simulink model "LCK_AVP"  (R2018b)
settings: Solver=FixedStepDiscrete  StartTime=0.0  StopTime=inf  FixedStep=0.01  RelTol=1e-3
PreLoadFcn:
  | if exist('tl_preloadfcn','file'), tl_preloadfcn(gcs,'4.4.0.41'); end
PostLoadFcn:
  | if any(exist('dsrtsu_mdlpostloadfcn', 'file') ~= 0), dsrtsu_mdlpostloadfcn('Execute', bdroot); end
  | if exist('tl_postloadfcn','file'), tl_postloadfcn(gcs,'4.4.0.41'); end
InitFcn:
  | if exist('tlds_init','file'), tlds_init(gcs); end
StartFcn:
  | if exist('tlds_start','file'), tlds_start(gcs); end
StopFcn:
  | if exist('tlds_stop','file'), tlds_stop(gcs); end
values from neighbouring files (symbols this model uses):
  C_DEG2RAD = 0.0175    [LCK_Macro.sldd]
  C_KPH2MPS = 0.2778    [LCK_Macro.sldd]
  C_NEARZERO = 0.0001    [LCK_Macro.sldd]
  C_ONE = 1.0    [LCK_Macro.sldd]
  C_RAD2DEG = 57.2958    [LCK_Macro.sldd]
  C_ZERO = 0.0    [LCK_Macro.sldd]
  k_accel_pedal_pos_per_speed_x : value not decoded    [LCK_LogicPara.sldd]
  k_accel_pedal_pos_per_speed_z : value not decoded    [LCK_LogicPara.sldd]
  k_brake_suprress_hold = 1000.0    [LCK_LogicPara.sldd]
  k_driver_appl_torque_filt = 50.0    [LCK_LogicPara.sldd]
  k_driver_suppression_hold_time = 3000.0    [LCK_LogicPara.sldd]
  k_hands_on_wheel_hold_msec = 500.0    [LCK_LogicPara.sldd]
  k_hands_on_wheel_torque_hi = 0.2    [LCK_LogicPara.sldd]
  k_hands_on_wheel_torque_lo = 0.15    [LCK_LogicPara.sldd]
  k_handsoff_delay_cycles = 50.0    [LCK_LogicPara.sldd]
  k_handsoff_torq_Lo_CR = 0.3    [LCK_LogicPara.sldd]
  k_handson_delay_cycles = 5.0    [LCK_LogicPara.sldd]
  k_HighAccel_suppress_hold = 3000.0    [LCK_LogicPara.sldd]
  k_HLR_suprress_hold = 3000.0    [LCK_LogicPara.sldd]
  k_hs_StrAng_CR_threshold_z : value not decoded    [LCK_LogicPara.sldd]
  k_LC_Exit_Switch = 0.0    [LCK_LogicPara.sldd]
  k_LCG_Configured = 1.0    [LCK_LogicPara.sldd]
  k_LCK_A0_Rdy2Act_UseConst = 0.0    [LCK_LogicPara.sldd]
  k_LCK_A0Fac_ActSta : value not decoded    [LCK_CtrlPara.sldd]
  k_LCK_A0Fac_DrvStm : value not decoded    [LCK_CtrlPara.sldd]
  k_LCK_A0Shift_LftCurv : value not decoded    [LCK_CtrlPara.sldd]
  k_LCK_A0Shift_RgtCurv : value not decoded    [LCK_CtrlPara.sldd]
  k_LCK_A0Shift_StraLan = 0.0    [LCK_CtrlPara.sldd]
  k_LCK_A0ShiftFac_Dy_LftCurv : value not decoded    [LCK_CtrlPara.sldd]
  k_LCK_A0ShiftFac_Dy_RgtCurv : value not decoded    [LCK_CtrlPara.sldd]
  k_LCK_A0ShiftFac_Vspd : value not decoded    [LCK_CtrlPara.sldd]
  k_LCK_accel_inhibit_thold = 35.0    [LCK_LogicPara.sldd]
  k_LCK_Active2Ready_Mask = 255.0    [LCK_LogicPara.sldd]
  k_LCK_CvatRateBks : value not decoded    [LCK_CtrlPara.sldd]
  k_LCK_CvatrBks : value not decoded    [LCK_CtrlPara.sldd]
  k_LCK_DFac_Dy : value not decoded    [LCK_CtrlPara.sldd]
  k_LCK_DFac_Dy_Curv : value not decoded    [LCK_CtrlPara.sldd]
  k_LCK_DFac_HaCurCen : value not decoded    [LCK_CtrlPara.sldd]
  k_LCK_DFac_HaCurSid : value not decoded    [LCK_CtrlPara.sldd]
  k_LCK_DFac_HadCurCen : value not decoded    [LCK_CtrlPara.sldd]
  k_LCK_DFac_HadCurSid : value not decoded    [LCK_CtrlPara.sldd]
  k_LCK_DFac_HadStrCen : value not decoded    [LCK_CtrlPara.sldd]
  k_LCK_DFac_HadStrSid : value not decoded    [LCK_CtrlPara.sldd]
  k_LCK_DFac_HaStrCen : value not decoded    [LCK_CtrlPara.sldd]
  k_LCK_DFac_HaStrSid : value not decoded    [LCK_CtrlPara.sldd]
  k_LCK_DFac_Rad : value not decoded    [LCK_CtrlPara.sldd]
  k_LCK_DFac_SA_CurCen : value not decoded    [LCK_CtrlPara.sldd]
  k_LCK_DFac_SA_CurSid : value not decoded    [LCK_CtrlPara.sldd]
  k_LCK_DFac_SA_StrCen : value not decoded    [LCK_CtrlPara.sldd]
  k_LCK_DFac_SA_StrSid : value not decoded    [LCK_CtrlPara.sldd]
  k_LCK_DFac_SS_CurCen : value not decoded    [LCK_CtrlPara.sldd]
  k_LCK_DFac_SS_CurSid : value not decoded    [LCK_CtrlPara.sldd]
  k_LCK_DFac_SS_StrCen : value not decoded    [LCK_CtrlPara.sldd]
  k_LCK_DFac_SS_StrSid : value not decoded    [LCK_CtrlPara.sldd]
  k_LCK_DFac_Vspd : value not decoded    [LCK_CtrlPara.sldd]
  k_LCK_DlyTm_DrvStim = 0.2    [LCK_CtrlPara.sldd]
  k_LCK_DTermMax = 2.0    [LCK_CtrlPara.sldd]
  k_LCK_DyBks_Curv : value not decoded    [LCK_CtrlPara.sldd]
  k_LCK_Enable_POOnly = 1.0    [LCK_LogicPara.sldd]
  k_LCK_Entry_DistBuffer = 0.1    [LCK_LogicPara.sldd]
  k_LCK_Fac_Vspd2RngThr_FalRec = 0.23    [LCK_CtrlPara.sldd]
  k_LCK_Ffw_CvatSwh = 0.0    [LCK_CtrlPara.sldd]
  k_LCK_Ffw_DyBks : value not decoded    [LCK_CtrlPara.sldd]
  k_LCK_Ffw_TimCon_CmdFlt = 0.0    [LCK_CtrlPara.sldd]
  k_LCK_FfwDeltaFac_Rad_Lft : value not decoded    [LCK_CtrlPara.sldd]
  k_LCK_FfwDeltaFac_Rad_Rgt : value not decoded    [LCK_CtrlPara.sldd]
  k_LCK_FfwDeltaFac_Vspd : value not decoded    [LCK_CtrlPara.sldd]
  k_LCK_FfwFac_CvatRate_Lft : value not decoded    [LCK_CtrlPara.sldd]
  k_LCK_FfwFac_CvatRate_Rgt : value not decoded    [LCK_CtrlPara.sldd]
  k_LCK_FfwFac_Dy : value not decoded    [LCK_CtrlPara.sldd]
  k_LCK_FfwFac_Rad_Lft : value not decoded    [LCK_CtrlPara.sldd]
  k_LCK_FfwFac_Rad_Rgt : value not decoded    [LCK_CtrlPara.sldd]
  k_LCK_FfwFac_Vspd : value not decoded    [LCK_CtrlPara.sldd]
  k_LCK_FfwTorq_Cvat : value not decoded    [LCK_CtrlPara.sldd]
  k_LCK_HAFac_ActSta : value not decoded    [LCK_CtrlPara.sldd]
  k_LCK_HAFac_DrvStm : value not decoded    [LCK_CtrlPara.sldd]
  k_LCK_HaloTime = 2000.0    [LCK_LogicPara.sldd]
  k_LCK_HaloTime_Switch = 0.0    [LCK_LogicPara.sldd]
  k_LCK_HARFac_ActSta : value not decoded    [LCK_CtrlPara.sldd]
  k_LCK_HARFac_DrvStm : value not decoded    [LCK_CtrlPara.sldd]
  k_LCK_Hed_DyBks : value not decoded    [LCK_CtrlPara.sldd]
  k_LCK_HedAngDiffX : value not decoded    [LCK_CtrlPara.sldd]
  k_LCK_HedAngRateDiffX : value not decoded    [LCK_CtrlPara.sldd]
  k_LCK_HndsOnWhel_DlyTm_Idl2Rdy = 0.0    [LCK_LogicPara.sldd]
  k_LCK_host_veh_width = 1.86    [LCK_LogicPara.sldd]
  k_LCK_Idle2Ready_Mask = 239.0    [LCK_LogicPara.sldd]
  k_LCK_Junc_SusTime = 1.0    [LCK_LogicPara.sldd]
  k_LCK_KpKdDecSlopeLmt = 10.0    [LCK_CtrlPara.sldd]
  k_LCK_KpKdIncSlopeLmt = 5.0    [LCK_CtrlPara.sldd]
  k_LCK_Lat_Ctrl_DFac_Lft = 1.0    [LCK_CtrlPara.sldd]
  k_LCK_Lat_Ctrl_DFac_Rgt = 1.05    [LCK_CtrlPara.sldd]
  k_LCK_Lat_Ctrl_Kd = 0.8    [LCK_CtrlPara.sldd]
  k_LCK_Lat_Ctrl_Ki = 0.5    [LCK_CtrlPara.sldd]
  k_LCK_Lat_Ctrl_Kp = 0.7    [LCK_CtrlPara.sldd]
  k_LCK_Lat_Ctrl_Kp_NearGain = 0.7    [LCK_CtrlPara.sldd]
  k_LCK_Lat_Ctrl_PFac_Lft = 1.0    [LCK_CtrlPara.sldd]
  k_LCK_Lat_Ctrl_PFac_Rgt = 1.05    [LCK_CtrlPara.sldd]
  k_LCK_Lat_Ctrl_TimCon_CmdFlt = 5.0    [LCK_CtrlPara.sldd]
  k_LCK_Lat_DFac_Rad : value not decoded    [LCK_CtrlPara.sldd]
  k_LCK_Lat_DFac_SS_Cur : value not decoded    [LCK_CtrlPara.sldd]
  k_LCK_Lat_DFac_SS_Str : value not decoded    [LCK_CtrlPara.sldd]
  k_LCK_Lat_DFac_Vspd : value not decoded    [LCK_CtrlPara.sldd]
  k_LCK_Lat_DyBks : value not decoded    [LCK_CtrlPara.sldd]
  k_LCK_Lat_IFac_Rad : value not decoded    [LCK_CtrlPara.sldd]
  k_LCK_Lat_IFac_Vspd : value not decoded    [LCK_CtrlPara.sldd]
  k_LCK_Lat_ILmtFac_Dy_CurvLan : value not decoded    [LCK_CtrlPara.sldd]
  k_LCK_Lat_ILmtFac_Dy_StraLan : value not decoded    [LCK_CtrlPara.sldd]
  k_LCK_Lat_ILmtFac_Rad : value not decoded    [LCK_CtrlPara.sldd]
  k_LCK_Lat_ILmtFac_Rad_NearGain = 1.0    [LCK_CtrlPara.sldd]
  k_LCK_Lat_ILmtFac_Vspd_CurvLan : value not decoded    [LCK_CtrlPara.sldd]
  k_LCK_Lat_ILmtFac_Vspd_StraLan : value not decoded    [LCK_CtrlPara.sldd]
  k_LCK_Lat_ITermLmt_Dy = 1.0    [LCK_CtrlPara.sldd]
  k_LCK_Lat_KpKdDecSlopeLmt = 10.0    [LCK_CtrlPara.sldd]
  k_LCK_Lat_KpKdIncSlopeLmt = 10.0    [LCK_CtrlPara.sldd]
  k_LCK_Lat_PFac_Dy_InnLftCur : value not decoded    [LCK_CtrlPara.sldd]
  k_LCK_Lat_PFac_Dy_InnRgtCur : value not decoded    [LCK_CtrlPara.sldd]
  k_LCK_Lat_PFac_Dy_OutLftCur : value not decoded    [LCK_CtrlPara.sldd]
  k_LCK_Lat_PFac_Dy_OutRgtCur : value not decoded    [LCK_CtrlPara.sldd]
  k_LCK_Lat_PFac_Dy_Str : value not decoded    [LCK_CtrlPara.sldd]
  k_LCK_Lat_PFac_Rad : value not decoded    [LCK_CtrlPara.sldd]
  ... (+153 more)
undefined symbols (not defined in the file or in its folder): k_LCK_CurvBks, K_LCK_SPA0A1A2_LMRngCmp_y
libraries: LateralControl_fcns_lib x58, simulink x24
(part 25 of 48)

== system LCK_AVP/Lateral_Control_Module/LCK_State_Ctrl/Det_Driver_Operation/Det_Driver_Steer_Override ==
  note: Pos = driver steers left
  note: Detect driver override during left lane marker intervention:
      | auto steer right + driver torque point left = f_driver_override
  note: Detect driver override during right lane marker intervention:
      | auto steer left + driver torque point right = f_driver_override
  note: Determine Driver Steering Override
  note: Steer angle rate: pos = velocity left
      | neg = velocity right
  note: Steer_angle: positive = left, CCW
      | negative= right,CW
  LCK_Mode : Inport  Description=_GWMAB30P4.LCK.000_38_
  Final_Torq_Cmd : Inport  Description=_GWMAB30P4.LCK.000_39_  Port=2
  Vspd : Inport  Description=_GWMAB30P4.LCK.000_38_  Port=3
  Steer_Torq : Inport  Description=_GWMAB30P4.LCK.000_38_  Port=4
  Add : Sum  Tag={'output',{'type','Float32'},'date',737395.45720195607}  Description=_GWMH9P3.LCK.000_11_  Inputs=-+
  Constant : Constant  Tag={'output',{'type','Int32'},'date',737237.63745600695}  Description=_GWMAB30P3.LCK.000_10_  Value=0
  Constant1 : Constant  Tag={'output',{'type','Int32'},'date',737237.63745672454}  Description=_GWMAB30P3.LCK.000_11_  Value=0
  Constant10 : Constant  Tag={'output',{'name','$P','class','EXTERN_CAL','type','Float32'},'date',737246.86422390048}  Description=_GWMAB30P2.LCK.000_1019_  Value=k_override_right_torq_thold
  Constant14 : Constant  Tag={'output',{'name','$P','class','EXTERN_CAL','type','Bool'},'date',737246.86427055555}  Description=_GWMAB30P2.LCK.000_1022_  Value=k_Ovrd_torq_thold_per_spd_sw
  Constant15 : Constant  Tag={'output',{'name','$P','class','EXTERN_CAL','type','Bool'},'date',737246.86427074077}  Description=_GWMAB30P2.LCK.000_1023_  Value=k_Ovrd_torq_thold_per_spd_sw
  Constant7 : Constant  Tag={'output',{'name','$P','class','EXTERN_CAL','type','Float32'},'date',737246.86422540504}  Description=_GWMAB30P2.LCK.000_1027_  Value=k_override_left_torq_thold
  Data Type Conversion1 : DataTypeConversion  Description=_GWMAB30P4.LCK.000_40_
  Data Type Conversion3 : DataTypeConversion  Description=_GWMAB30P4.LCK.000_41_
  Data Type Conversion4 : DataTypeConversion  Description=_GWMAB30P4.LCK.000_42_
  Data Type Conversion8 : DataTypeConversion  Description=_GWMAB30P4.LCK.000_43_
  Delay : Delay  DelayLength=1  InitialCondition=0
  Delay1 : Delay  DelayLength=1  InitialCondition=0
  Gain : Gain  Tag={'output',{'type','Float32'},'gain',{'type','Int32'},'date',737189.64304143516}  Description=_GWMAB30P2.LCK.000_1028_  Gain=-1
  Logical Operator : Logic  Tag={'date',737237.63745719905}  Description=_GWMAB30P3.LCK.000_12_  AllPortsSameDT=off  OutDataTypeStr=boolean
  Logical Operator1 : Logic  Tag={'date',737237.63745734957}  Description=_GWMAB30P3.LCK.000_13_  AllPortsSameDT=off  OutDataTypeStr=boolean
  Logical Operator2 : Logic  Tag={'date',737393.53532744211}  Description=_GWMH9P3.LCK.000_12_  Operator=OR  AllPortsSameDT=off  OutDataTypeStr=boolean
  Relational Operator : RelationalOperator  Tag={'date',737237.63745749998}  Description=_GWMAB30P3.LCK.000_14_  Operator=<  OutDataTypeStr=boolean  RndMeth=Nearest
  Relational Operator1 : RelationalOperator  Tag={'date',737237.63745763886}  Description=_GWMAB30P3.LCK.000_15_  Operator=>  OutDataTypeStr=boolean  RndMeth=Nearest
  Relational Operator3 : RelationalOperator  Tag={'date',737184.60396784719}  Description=_GWMAB30P2.LCK.000_1039_  OutDataTypeStr=boolean  RndMeth=Nearest
  Relational Operator6 : RelationalOperator  Tag={'date',737184.60396796302}  Description=_GWMAB30P2.LCK.000_1040_  Operator=<=  OutDataTypeStr=boolean  RndMeth=Nearest
  Right_distance_sustain_period : Stateflow chart  Description=_GWMAB30P4.LCK.000_44_  TreatAsAtomicUnit=on
  Switch : Switch  Tag={'output',{'inheritscaling',1},'threshold',{'type','Int32','scalar',1},'date',737395.45749100694}  Description=_GWMH9P3.LCK.000_13_  Criteria=u2 ~= 0
  Switch2 : Switch  Tag={'output',{'inheritscaling',1},'threshold',{'type','Int32','scalar',1},'date',737189.6437576852}  Description=_GWMAB30P2.LCK.000_1045_  Threshold=0.5
  Switch3 : Switch  Tag={'output',{'inheritscaling',1},'threshold',{'type','Int32','scalar',1},'date',737189.64308021986}  Description=_GWMAB30P2.LCK.000_1046_  Threshold=0.5
  Unit Delay1 : UnitDelay  Tag={'output',{'inheritscaling',1},'state',{'type','Int32'},'date',737395.45284084487}  Description=_GWMH9P3.LCK.000_14_  SampleTime=-1
  Unit Delay2 : UnitDelay  Tag={'output',{'inheritscaling',1},'state',{'type','Int32'},'date',737395.45284105325}  Description=_GWMH9P3.LCK.000_15_  SampleTime=-1
  k_LCK_Ovrd_Torq_Hys : Constant  Tag={'output',{'name','$P','class','EXTERN_CAL','type','Float32'},'date',737395.45723880793}  Description=_GWMH9P3.LCK.000_16_  Value=k_LCK_Ovrd_Torq_Hys
  k_LCK_ovrd_torq_thold_per_spd : Lookup_n-D  Tag={'input',{'name','$P','class','EXTERN_CAL','type','Float32'},'output',{'type','Float32'},'table',{'name','$P','class','EXTERN_CAL','type','Float32'},'date',737237.77625888889}  Description=_GWMAB30P2.LCK.000_1047_  NumberOfTableDimensions=1  BreakpointsForDimension1=k_LCK_ovrd_torq_thold_per_spd_x  IndexSearchMethod=Linear search  Table=k_LCK_ovrd_torq_thold_per_spd_z  ExtrapMethod=Clip  InputSameDT=on
  left_distance_sustain_period : Stateflow chart  Description=_GWMAB30P4.LCK.000_49_  TreatAsAtomicUnit=on
  within_distance_sustain_period : Constant  Tag={'output',{'name','$P','class','EXTERN_CAL','type','UInt16'},'date',737246.8642231134}  Description=_GWMAB30P2.LCK.000_1051_  Value=k_override_torq_sustain_period
  within_distance_sustain_period1 : Constant  Tag={'output',{'name','$P','class','EXTERN_CAL','type','UInt16'},'date',737246.86422331014}  Description=_GWMAB30P2.LCK.000_1052_  Value=k_override_torq_sustain_period
  f_driver_override_left_trq : Outport  Description=_GWMAB30P4.LCK.000_54_
  f_driver_override_right_trq : Outport  Description=_GWMAB30P4.LCK.000_54_  Port=2
  wires:
  within_distance_sustain_period1/1 -> Right_distance_sustain_period/2(k_override_torq_sustain_period)
  Constant14/1 -> Switch2/2
  Vspd/1 -> [IP_veh_spd_kph]
  [IP_veh_spd_kph] -> k_LCK_ovrd_torq_thold_per_spd/1
  Unit Delay2/1 -> Logical Operator2/2
  Constant1/1 -> Relational Operator1/2
  Constant/1 -> Relational Operator/2
  k_LCK_Ovrd_Torq_Hys/1 -> Add/1
  Data Type Conversion4/1 -> [f_driver_override_right_trq], f_driver_override_right_trq/1
  k_LCK_ovrd_torq_thold_per_spd/1 -> Add/2, Switch/3
  Data Type Conversion3/1 -> [f_driver_override_left_trq], f_driver_override_left_trq/1
  Relational Operator6/1 -> Data Type Conversion1/1
  [driver_applied_torque_filt] -> Relational Operator6/1
  within_distance_sustain_period/1 -> left_distance_sustain_period/2(k_override_torq_sustain_period)
  Unit Delay1/1 -> Logical Operator2/1
  [LCK_Mode] -> left_distance_sustain_period/3(LCK_Mode)
  [driver_applied_torque_filt] -> Relational Operator3/1
  left_distance_sustain_period/1(sustain_value_out) -> Logical Operator/2
  Switch3/1 -> Relational Operator6/2
  Constant15/1 -> Switch3/2
  Relational Operator3/1 -> Data Type Conversion8/1
  LCK_Mode/1 -> Delay1/1
  Constant7/1 -> Switch2/3
  Switch2/1 -> Relational Operator3/2
  Gain/1 -> Switch3/1
  Relational Operator/1 -> Logical Operator/1
  Add/1 -> Switch/1
  Logical Operator/1 -> Data Type Conversion3/1
  Relational Operator1/1 -> Logical Operator1/1
  Constant10/1 -> Switch3/3
  Final_Torq_Cmd/1 -> Delay/1
  [f_driver_override_left_trq] -> Unit Delay1/1
  Switch/1 -> Switch2/1, Gain/1
  Right_distance_sustain_period/1(sustain_value_out) -> Logical Operator1/2
  [f_driver_override_right_trq] -> Unit Delay2/1
  [LCK_Mode] -> Right_distance_sustain_period/3(LCK_Mode)
  [Final_Torq_n_1_LCK] -> Relational Operator1/1
  [Final_Torq_n_1_LCK] -> Relational Operator/1
  Data Type Conversion1/1 -> Right_distance_sustain_period/1(current_input)
  Logical Operator2/1 -> Switch/2
  Data Type Conversion8/1 -> left_distance_sustain_period/1(current_input)
  Logical Operator1/1 -> Data Type Conversion4/1
  Steer_Torq/1 -> [driver_applied_torque_filt]
  Delay/1 -> [Final_Torq_n_1_LCK]
  Delay1/1 -> [LCK_Mode]
